simulink model "t4_2_Atractor_de_Lorenz"  (R2024a)
settings: Solver=ode4  StartTime=0.0  StopTime=100  FixedStep=.01  RelTol=1e-3
InitFcn:
  | sigma = 10;
  | rho = 28;
  | beta = 8/3;
settings Model: Creator=jibmo  LastModifiedBy=scpmoxxa
settings DataIOCC: SaveFormat=Array
settings OptimizationCC: ReuseModelBlockBuffer=off
settings RTWCC: GPUComputeCapability=3.5

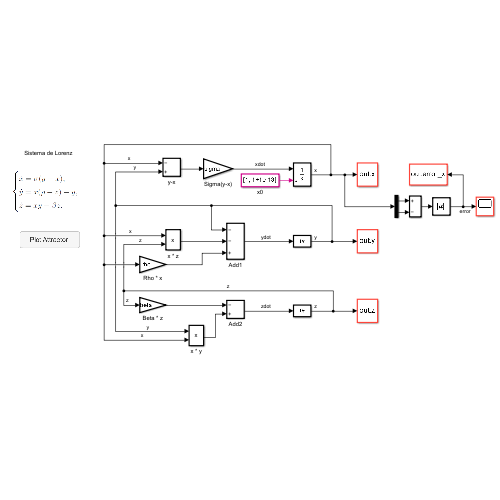
[thumbnail: Simulink's stored preview of the top-level diagram]
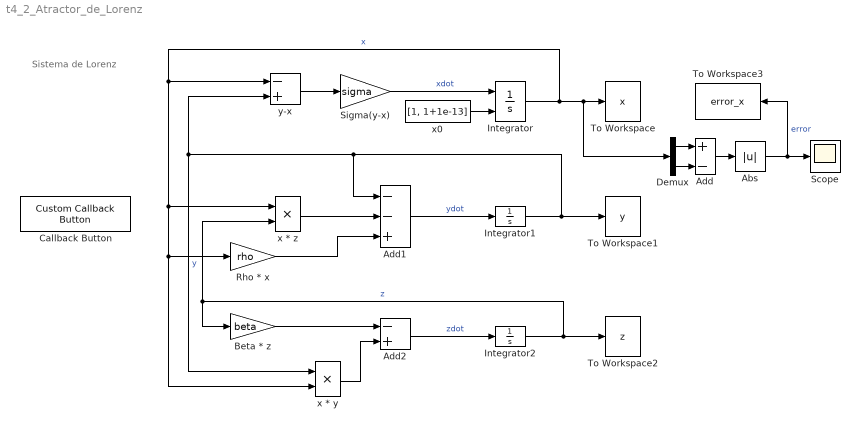
== system t4_2_Atractor_de_Lorenz ==
  note: Sistema de Lorenz
  Abs : Abs  SaturateOnIntegerOverflow=off
  Add : Sum  Inputs=+-
  Add1 : Sum  Inputs=--+
  Add2 : Sum  Inputs=-+
  Beta * z : Gain  Gain=beta  SaturateOnIntegerOverflow=on  OutDataTypeStr=Inherit: Same as input  ParamDataTypeStr=Inherit: Same as input
  Callback Button : CustomCallbackButton  Configuration="{\"components\":[{\"name\":\"BackgroundImageComponent\",\"settings\":{\"image\":{\"size\":[0,0],\"src\":\"default\",\"srcOrientation\":\"Right\"},\"position\":[0,0,1,1]}},{\"name\":\"ButtonStateComponent\",\"settings\":{\"buttonType\":\"momentary\",\"clickFcn\":\"close all\\n\\nfigure;\\nplot3(out.x,out.y,out.z);\\ntitle('Atractor de Lorenz');\\nxlabel('x');zlabel('z');ylabel('y');\\n\\nfigure;\\nplot(out.tout,[out.x,out.y,out.z]);\\nxlabel('t')\\nylabel('x,y,z')\\n\\nfigure;\\nloglog(out.tout,(out.error_x))\\nxlabel('t')\\nylabel('Error en x')\\n\\nfigure;\\ndt = 0.01;\\nplot(out.tout(15\\/dt:50\\/dt),log(out.error_x(15\\/dt:50\\/dt)))\\nxlabel('t')\\nylabel('Logaritmo del error en x')\\n\\n\",\"onValue\":1,\"position\":[0,0,1,1],\"pressDelay\":\"500\",\"pressFcn\":\"\",\"repeatInterval\":\"0\",\"states\":[{\"horizontalAlignment\":\"center\",\"image\":{\"position\":[0,0,1,1],\"src\":\"default\",\"srcOrientation\":\"Right\"},\"label\":{\"color\":[0.01176470588,0.01176470588,0.01176470588,1],\"icon\":{\"size\":[0,0],\"src\":\"default\",\"srcOrientation\":\"Right\"},\"iconPlacement\":\"left\",\"text\":{\"content\":\"Plot Attractor\"}},\"labelOffset\":[0,0],\"verticalAlignment\":\"middle\"},{\"horizontalAlignment\":\"center\",\"image\":{\"position\":[0,0,1,1],\"src\":\"default\",\"srcOrientation\":\"Right\"},\"label\":{\"color\":[0.01176470588,0.01176470588,0.01176470588,1],\"icon\":{\"size\":[0,0],\"src\":\"default\",\"srcOrientation\":\"Right\"},\"iconPlacement\":\"left\",\"text\":{\"content\":\"Plot Attractor\"}},\"labelOffset\":[0,0],\"verticalAlignment\":\"middle\"},{\"horizontalAlignment\":\"center\",\"image\":{\"position\":[0,0,1,1],\"src\":\"default\",\"srcOrientation\":\"Right\"},\"label\":{\"color\":[0.01176470588,0.01176470588,0.01176470588,1],\"icon\":{\"size\":[0,0],\"src\":\"default\",\"srcOrientation\":\"Right\"},\"iconPlacement\":\"left\",\"text\":{\"content\":\"Plot Attractor\"}},\"labelOffset\":[0,0],\"verticalAlignment\":\"middle\"},{\"horizontalAlignment\":\"center\",\"image\":{\"position\":[0,0,1,1],\"src\":\"default\",\"srcOrientation\":\"Right\"},\"label\":{\"color\":[0.01176470588,0.01176470588,0.01176470588,1],\"icon\":{\"size\":[0,0],\"src\":\"default\",\"srcOrientation\":\"Right\"},\"iconPlacement\":\"left\",\"text\":{\"content\":\"Plot Attractor\"}},\"labelOffset\":[0,0],\"verticalAlignment\":\"middle\"}]}},{\"name\":\"ForegroundImageComponent\",\"settings\":{\"image\":{\"size\":[0,0],\"src\":\"default\",\"srcOrientation\":\"Right\"},\"isForeground\":1,\"position\":[0,0,1,1]}}],\"settings\":{\"BindingType\":\"standalone\",\"backgroundColor\":[244,244,244,1],\"backgroundOffset\":0.2,\"backgroundOpacity\":1,\"fixedAspectRatio\":\"off\",\"foregroundColor\":[0.01176470588,0.01176470588,0.01176470588,1],\"migratedFromLegacy\":true,\"useBackgroundColor\":true,\"variant\":\"callback\",\"version\":\"R2023a\"},\"type\":\"Button\"}"  CustomBackgroundColor="{\"color\":[0.9568627451,0.9568627451,0.9568627451],\"show\":true}"
  Demux : Demux  Outputs=2
  Integrator : Integrator  InitialConditionSource=external  InitialCondition=1
  Integrator1 : Integrator  InitialCondition=1
  Integrator2 : Integrator  InitialCondition=1
  Rho * x : Gain  Gain=rho  SaturateOnIntegerOverflow=on  OutDataTypeStr=Inherit: Same as input  ParamDataTypeStr=Inherit: Same as input
  Scope : Scope
  Sigma(y-x) : Gain  Gain=sigma  SaturateOnIntegerOverflow=on  OutDataTypeStr=Inherit: Same as input  ParamDataTypeStr=Inherit: Same as input
  To Workspace : ToWorkspace  VariableName=x  SampleTime=-1
  To Workspace1 : ToWorkspace  VariableName=y  SampleTime=-1
  To Workspace2 : ToWorkspace  VariableName=z  SampleTime=-1
  To Workspace3 : ToWorkspace  VariableName=error_x  SampleTime=-1
  x * y : Product  InputSameDT=on  RndMeth=Zero  SaturateOnIntegerOverflow=on  OutDataTypeStr=Inherit: Same as first input
  x * z : Product  InputSameDT=on  RndMeth=Zero  SaturateOnIntegerOverflow=on  OutDataTypeStr=Inherit: Same as first input
  x0 : Constant  Value=[1, 1+1e-13]
  y-x : Sum  Inputs=-+
  wires:
  Integrator1/1 -> x * y/1, y-x/2, Add1/1, To Workspace1/1  "y"
  y-x/1 -> Sigma(y-x)/1
  Sigma(y-x)/1 -> Integrator/1  "xdot"
  Integrator2/1 -> x * z/2, Beta * z/1, To Workspace2/1  "z"
  Integrator/1 -> Demux/1, To Workspace/1, y-x/1, x * z/1, x * y/2, Rho * x/1  "x"
  Add1/1 -> Integrator1/1  "ydot"
  Rho * x/1 -> Add1/3
  x * z/1 -> Add1/2
  Add2/1 -> Integrator2/1  "zdot"
  Beta * z/1 -> Add2/1
  x * y/1 -> Add2/2
  x0/1 -> Integrator/2
  Add/1 -> Abs/1
  Abs/1 -> To Workspace3/1, Scope/1  "error"
  Demux/1 -> Add/1
  Demux/2 -> Add/2
